simulink model "UPQC"  (R2021b)
settings: Solver=ode23tb  StartTime=0.0  StopTime=2.5  RelTol=1e-6  EnableMultiTasking=on
InitFcn:
  | Ts=20e-6;
undefined symbols (not defined in the file): DiscIntNeverNeededParam
libraries: spsIGBTDiodeLib x12, spsDiodeLib x6, spsSeriesRLCBranchLib x5, powerlib_extras x3, spsThreePhaseVIMeasurementLib x3, spsSaturableTransformerLib x3, spsThreePhaseSeriesRLCBranchLib x2, spsVoltageMeasurementLib x1, spsMultimeterLib x1, spsThreePhaseProgrammableVoltageSourceLib x1, spsGroundLib x1, spspowerguiLib x1
settings Model: Creator=srikanth  LastModifiedBy=B Sai Soumath
settings SolverCC: AlgebraicLoopSolver=LineSearch
settings DataIOCC: LimitDataPoints=on  SaveFormat=Array  SignalLoggingSaveFormat=ModelDataLogs  SaveOutput=off  SaveTime=off  ReturnWorkspaceOutputs=off
settings OptimizationCC: ExpressionDepthLimit=2147483647  LifeSpan=inf
settings DebuggingCC: AlgebraicLoopMsg=none  UnderspecifiedInitializationDetection=Classic  MergeDetectMultiDrivingBlocksExec=none  SolverPrmCheckMsg=warning  FcnCallInpInsideContextMsg=warning  StateNameClashWarn=warning  SFUnexpectedBacktrackingDiag=warning  SFNoUnconditionalDefaultTransitionDiag=warning  SFExecutionAtInitializationDiag=none  SFMachineParentedDataDiag=warning  ArithmeticOperatorsInVariantConditions=warning
settings HardwareCC: ProdBitPerPointer=32  ProdBitPerSizeT=32  ProdBitPerPtrDiffT=32  ProdLargestAtomicFloat=None  ProdIntDivRoundTo=Undefined  ProdEndianess=Unspecified  ProdWordSize=32  ProdHWDeviceType=32-bit Generic
settings ModelReferenceCC: PropagateSignalLabelsOutOfModel=off
settings SFSimCC: SimUseLocalCustomCode=off  CustomCodeUndefinedFunction=UseInterfaceOnly
settings RTWCC: RTWUseLocalCustomCode=off
settings CodeAppCC: StateflowObjectComments=on
settings GRTTargetCC: TargetLangStandard=C89/C90 (ANSI)  CombineOutputUpdateFcns=off  GRTInterface=on
settings ConfigComp: CovMetricSettings=dw  CovSaveCumulativeToWorkspaceVar=on  CovSaveSingleToWorkspaceVar=on  CovExternalEMLEnable=off

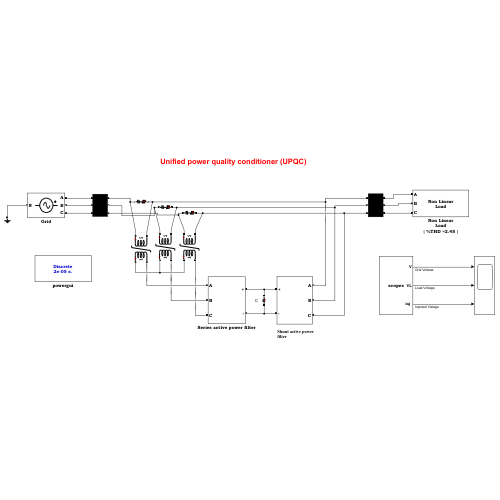
[thumbnail: Simulink's stored preview of the top-level diagram]
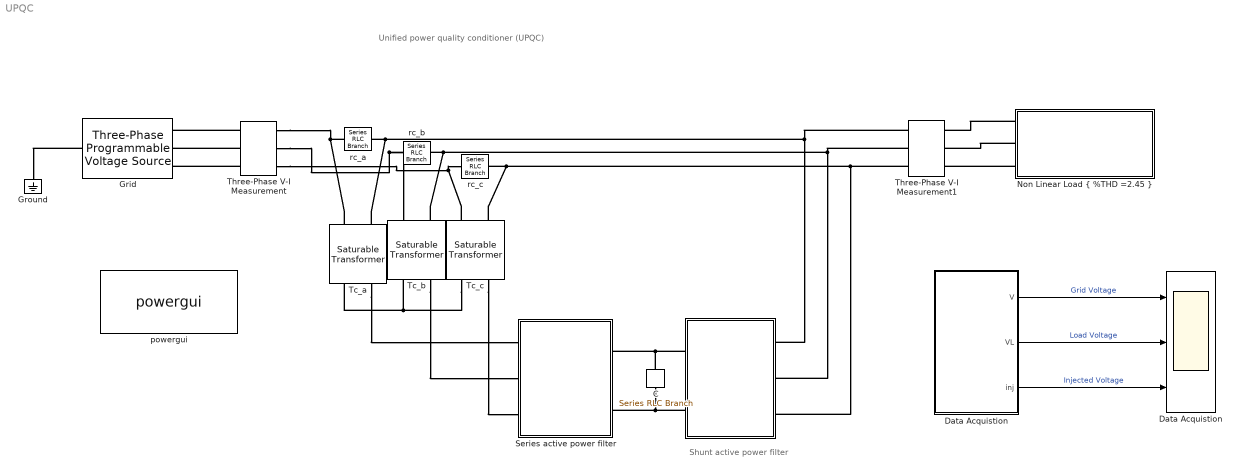
== system UPQC ==
  note: Shunt active power filter
  note: Unified power quality conditioner (UPQC)
  "                  " : Subsystem
  C : spsSeriesRLCBranchLib/Series RLC Branch  LConnTagsString=__new0  RConnTagsString=__new0  BranchType=C  Resistance=1  Inductance=1e-3  SetiL0=off  InitialCurrent=0  Capacitance=100e-6  Setx0=off  InitialVoltage=700  Measurements=None
  Data Acquistion : Scope  NumInputPorts=3
  Data Acquistion : Subsystem
      mask Display: fprintf('scopes')
  Grid : spsThreePhaseProgrammableVoltageSourceLib/Three-Phase Programmable Voltage Source  PositiveSequence="[400  0 50]"  VariationEntity=Amplitude  VariationType=Table of time-amplitude pairs  VariationTypeAlt=Step  VariationStep=0.5  VariationRate=10  VariationMagnitude=0.3  VariationFrequency=2  VariationTiming=[1 2]  VariationPhaseA=off  Amplitudes=[1 0.7 1 1.3 1]  TimeValues=[0 0.9 1 1.6 1.7]  HarmonicGeneration=on  HarmonicA=[5 0.2 0 2]  HarmonicB=[7 0.05 0 1]  Timing=[0.3 0.4]  BusType=swing  Pref=0  Qref=0  Qmin=-inf  Qmax=inf
  Ground : spsGroundLib/Ground  LConnTagsString=a
  "Non Linear Load { %THD =2.45 }" : Subsystem
      mask Display: fprintf('Non Linear\nLoad')
  Series active power filter : Subsystem
  Tc_a : spsSaturableTransformerLib/Saturable Transformer  ThreeWindings=off  Hysteresis=off  DataFile='hysteresis.mat'  Measurements=None  UNITS=pu  NominalPower=[4000 50]  Winding1="[380  0.02  0.02 ]"  Winding2="[380  0.02  0.02]"  Winding3="[ 315e3  0.002  0.08 ]"  Saturation=[ 0 0 ;1.016 9.043]*1e-3  CoreLoss=[117 0]  BreakLoop=off  DiscreteSolver=Trapezoidal iterative  DataType=off  InitialFlux=0  TransfoNumber=1
      settings: SourceProductBaseCode=PS
  Tc_b : spsSaturableTransformerLib/Saturable Transformer  ThreeWindings=off  Hysteresis=off  DataFile='hysteresis.mat'  Measurements=None  UNITS=pu  NominalPower=[4000 50]  Winding1="[380  0.02  0.02 ]"  Winding2="[380  0.02  0.02]"  Winding3="[ 315e3  0.002  0.08 ]"  Saturation=[ 0 0 ;1.016 9.043]*1e-3  CoreLoss=[117 0]  BreakLoop=off  DiscreteSolver=Trapezoidal iterative  DataType=off  InitialFlux=0  TransfoNumber=1
      settings: SourceProductBaseCode=PS
  Tc_c : spsSaturableTransformerLib/Saturable Transformer  ThreeWindings=off  Hysteresis=off  DataFile='hysteresis.mat'  Measurements=None  UNITS=pu  NominalPower=[4000 50]  Winding1="[380  0.02  0.02 ]"  Winding2="[380  0.02  0.02]"  Winding3="[ 315e3  0.002  0.08 ]"  Saturation=[ 0 0 ;1.016 9.043]*1e-3  CoreLoss=[117 0]  BreakLoop=off  DiscreteSolver=Trapezoidal iterative  DataType=off  InitialFlux=0  TransfoNumber=1
      settings: SourceProductBaseCode=PS
  Three-Phase V-I Measurement : spsThreePhaseVIMeasurementLib/Three-Phase V-I Measurement  VoltageMeasurement=phase-to-ground  SetLabelV=on  LabelV=Vabc  Vpu=off  VpuLL=off  CurrentMeasurement=yes  SetLabelI=on  LabelI=Iabc  Ipu=off  Pbase=100e6  Vbase=500e3  OutputType=Complex  PhasorSimulation=off  PSBequivalent=0
  Three-Phase V-I Measurement1 : spsThreePhaseVIMeasurementLib/Three-Phase V-I Measurement  VoltageMeasurement=phase-to-ground  SetLabelV=on  LabelV=V_L  Vpu=off  VpuLL=off  CurrentMeasurement=yes  SetLabelI=on  LabelI=I_L  Ipu=off  Pbase=100e6  Vbase=500e3  OutputType=Complex  PhasorSimulation=off  PSBequivalent=0
  powergui : spspowerguiLib/powergui  Priority=1  SimulationMode=Discrete  SampleTime=Ts  frequency=60  Iterations=50  frequencyindice=50  Pbase=100e6  ErrMax=1e-4  UnitsV=kV  UnitsW=MW  buscounter=0  FunctionMessages=off  echomessages=off  EnableUseOfTLC=off  CurrentSourceSwitches=off  DisableSnubberDevices=off  DisableRonSwitches=off  DisableVfSwitches=off  DisplayEquations=off  AutomaticDiscreteSolvers=off  SolverType=Tustin/Backward Euler (TBE)  Interpol=off  ExternalGateDelay=off  methode=off  Ts=0  x0status=blocks  SPID=off  SwTol=0  HookPort=off  NonlinearTolerance=1e-4  nMaxIteration=100  ContinueOnMaxIteration=off  RestoreLinks=warning  ResistiveCurrentMeasurement=off  Frange=[0:2:500]  Ylog=off  Xlog=on  ShowGrid=off  save=off  variable=ZData  structure=Grid_pi  ZoomFFT=on  StartTime=0.9  cycles=1  DisplayStyle=3  fundamental=50  FreqAxis=on  MaxFrequency=2500  frequencyindicesteady=1  RmsSteady=1  display=off
  rc_a : spsSeriesRLCBranchLib/Series RLC Branch  LConnTagsString=__new0  RConnTagsString=__new0  BranchType=RC  Resistance=1  Inductance=1e-3  SetiL0=off  InitialCurrent=0  Capacitance=100e-6  Setx0=off  InitialVoltage=0  Measurements=Branch voltage
  rc_b : spsSeriesRLCBranchLib/Series RLC Branch  LConnTagsString=__new0  RConnTagsString=__new0  BranchType=RC  Resistance=1  Inductance=1e-3  SetiL0=off  InitialCurrent=0  Capacitance=100e-6  Setx0=off  InitialVoltage=0  Measurements=Branch voltage
  rc_c : spsSeriesRLCBranchLib/Series RLC Branch  LConnTagsString=__new0  RConnTagsString=__new0  BranchType=RC  Resistance=1  Inductance=1e-3  SetiL0=off  InitialCurrent=0  Capacitance=100e-6  Setx0=off  InitialVoltage=0  Measurements=Branch voltage
  wires:
  Data Acquistion/1(V) -> Data Acquistion/1  "Grid Voltage"
  Data Acquistion/2(VL) -> Data Acquistion/2  "Load Voltage"
  Data Acquistion/3("inj ") -> Data Acquistion/3  "Injected Voltage"
  connections:
  Grid/LConn1 -- Ground/LConn1
  Three-Phase V-I Measurement/LConn1 -- Grid/RConn1
  Three-Phase V-I Measurement/LConn2 -- Grid/RConn2
  Three-Phase V-I Measurement/LConn3 -- Grid/RConn3
  rc_a/RConn1 -- Three-Phase V-I Measurement/RConn1 -- Tc_a/RConn1
  rc_b/RConn1 -- Three-Phase V-I Measurement/RConn2 -- Tc_b/RConn1
  Three-Phase V-I Measurement/RConn3 -- rc_c/RConn1 -- Tc_c/RConn1
  Tc_a/LConn2 -- Series active power filter/LConn1
  Tc_b/LConn2 -- Series active power filter/LConn2
  Tc_c/LConn2 -- Series active power filter/LConn3
  Tc_c/LConn1 -- Tc_a/LConn1 -- Tc_b/LConn1
  "                  "/RConn2 -- C/RConn1 -- Series active power filter/RConn2
  Three-Phase V-I Measurement1/LConn3 -- "                  "/LConn3 -- Tc_c/RConn2 -- rc_c/LConn1
  Three-Phase V-I Measurement1/LConn2 -- "                  "/LConn2 -- Tc_b/RConn2 -- rc_b/LConn1
  Three-Phase V-I Measurement1/LConn1 -- "                  "/LConn1 -- Tc_a/RConn2 -- rc_a/LConn1
  "                  "/RConn1 -- C/LConn1 -- Series active power filter/RConn1
  "Non Linear Load { %THD =2.45 }"/LConn1 -- Three-Phase V-I Measurement1/RConn1
  "Non Linear Load { %THD =2.45 }"/LConn2 -- Three-Phase V-I Measurement1/RConn2
  "Non Linear Load { %THD =2.45 }"/LConn3 -- Three-Phase V-I Measurement1/RConn3

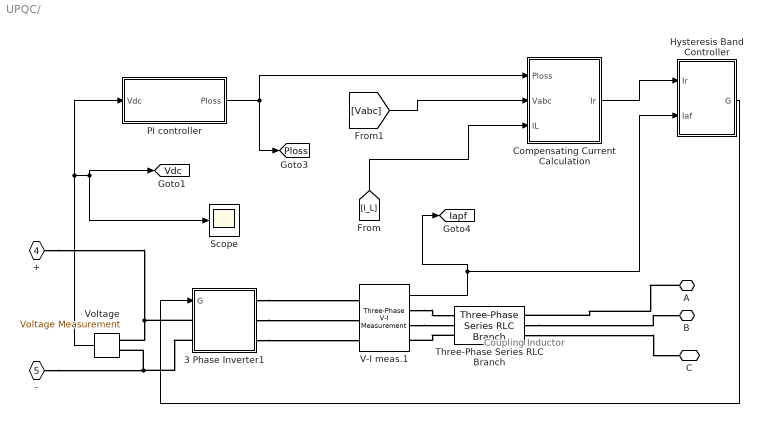
== system UPQC/                   ==
  note: Coupling Inductor
  3 Phase Inverter1 : Subsystem
  Compensating Current Calculation : Subsystem
  Hysteresis Band Controller : Subsystem
  PI controller : Subsystem
  Scope : Scope
  Three-Phase Series RLC Branch : spsThreePhaseSeriesRLCBranchLib/Three-Phase Series RLC Branch  LConnTagsString=A|B|C  RConnTagsString=A|B|C  BranchType=L  Resistance=0.0001  Inductance=10e-3  Capacitance=.2e-3  Measurements=None
  V-I meas.1 : spsThreePhaseVIMeasurementLib/Three-Phase V-I Measurement  VoltageMeasurement=phase-to-ground  SetLabelV=on  LabelV=Vnm  Vpu=off  VpuLL=off  CurrentMeasurement=yes  SetLabelI=off  LabelI=Iabc  Ipu=off  Pbase=100e6  Vbase=500e3  OutputType=Complex  PhasorSimulation=off  PSBequivalent=0
  Voltage : spsVoltageMeasurementLib/Voltage Measurement  PhasorSimulation=off  OutputType=Complex  PSBequivalent=0
  A : PMIOPort  Side=Left
  B : PMIOPort  Port=2  Side=Left
  C : PMIOPort  Port=3  Side=Left
  + : PMIOPort  Tag=PMCPort  Port=4  Side=Right
  - : PMIOPort  Tag=PMCPort  Port=5  Side=Right
  tag scope: Iapf=global, Ploss=global, Vdc=global
  wires:
  V-I meas.1/1 -> Hysteresis Band Controller/2(Iaf), [Iapf]
  Voltage/1 -> PI controller/1(Vdc), Scope/1, [Vdc]
  [I_L] -> Compensating Current Calculation/3(IL)
  [Vabc] -> Compensating Current Calculation/2(Vabc)
  Compensating Current Calculation/1(Ir) -> Hysteresis Band Controller/1(Ir)
  PI controller/1(Ploss) -> [Ploss], Compensating Current Calculation/1(Ploss)
  Hysteresis Band Controller/1(G) -> 3 Phase Inverter1/1(G)
  connections:
  +/RConn1 -- 3 Phase Inverter1/LConn1 -- Voltage/LConn1
  3 Phase Inverter1/RConn1 -- V-I meas.1/LConn1
  3 Phase Inverter1/RConn2 -- V-I meas.1/LConn2
  Three-Phase Series RLC Branch/LConn3 -- V-I meas.1/RConn3
  V-I meas.1/RConn2 -- Three-Phase Series RLC Branch/LConn2
  3 Phase Inverter1/RConn3 -- V-I meas.1/LConn3
  V-I meas.1/RConn1 -- Three-Phase Series RLC Branch/LConn1
  A/RConn1 -- Three-Phase Series RLC Branch/RConn1
  Three-Phase Series RLC Branch/RConn2 -- B/RConn1
  Three-Phase Series RLC Branch/RConn3 -- C/RConn1
  -/RConn1 -- 3 Phase Inverter1/LConn2 -- Voltage/LConn2

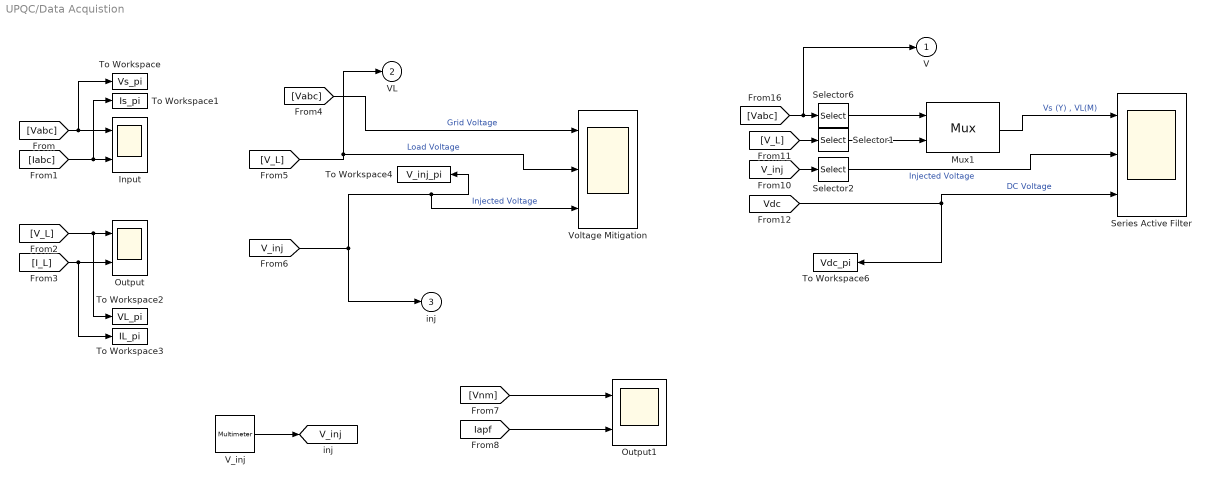
== system UPQC/Data Acquistion ==
  Input : Scope  NumInputPorts=2
  Mux1 : Mux  Inputs=2
      settings: DisplayOption=signals
  Output : Scope  NumInputPorts=2
  Output1 : Scope  NumInputPorts=2
  Selector1 : Selector  InputPortWidth=3  IndexOptions=Index vector (dialog)  Indices=1  OutputSizes=1
  Selector2 : Selector  InputPortWidth=3  IndexOptions=Index vector (dialog)  Indices=1  OutputSizes=1
  Selector6 : Selector  InputPortWidth=3  IndexOptions=Index vector (dialog)  Indices=1  OutputSizes=1
  Series Active Filter : Scope  NumInputPorts=3
  To Workspace : ToWorkspace  VariableName=Vs_pi  SampleTime=Ts
  To Workspace1 : ToWorkspace  VariableName=Is_pi  SampleTime=Ts
  To Workspace2 : ToWorkspace  VariableName=VL_pi  SampleTime=Ts
  To Workspace3 : ToWorkspace  VariableName=IL_pi  SampleTime=Ts
  To Workspace4 : ToWorkspace  VariableName=V_inj_pi  SampleTime=Ts
  To Workspace6 : ToWorkspace  VariableName=Vdc_pi  SampleTime=Ts
  V_inj : spsMultimeterLib/Multimeter  PhasorSimulation=off  OutputType=Complex  sel=[1 2 3]  L=3  Gain=[1 1 1]  yselected={'Ub: rc_a','Ub: rc_b','Ub: rc_c'};  PSBOutputType=1  PSBequivalent=0  AxesSetting=[0,0.1,-100,100]  Display=0  SavedBlockNames=-11
  Voltage Mitigation : Scope  NumInputPorts=3
  V : Outport  VectorParamsAs1DForOutWhenUnconnected=off
  VL : Outport  Port=2  VectorParamsAs1DForOutWhenUnconnected=off
  "inj " : Outport  Port=3  VectorParamsAs1DForOutWhenUnconnected=off
  tag scope: V_inj=global
  wires:
  [Vabc] -> Input/1, To Workspace/1
  [Iabc] -> Input/2, To Workspace1/1
  [V_L] -> Output/1, To Workspace2/1
  [I_L] -> Output/2, To Workspace3/1
  [Vabc] -> Voltage Mitigation/1  "Grid Voltage"
  [V_L] -> Voltage Mitigation/2, VL/1  "Load Voltage"
  [V_inj] -> Voltage Mitigation/3, To Workspace4/1, "inj "/1  "Injected Voltage"
  [V_L] -> Selector1/1
  [V_inj] -> Selector2/1
  [Vdc] -> Series Active Filter/3, To Workspace6/1  "DC Voltage"
  Selector2/1 -> Series Active Filter/2  "Injected Voltage"
  [Vabc] -> Selector6/1, V/1
  Selector1/1 -> Mux1/2
  Mux1/1 -> Series Active Filter/1  "Vs (Y) , VL(M)"
  Selector6/1 -> Mux1/1
  V_inj/1 -> [V_inj]
  [Iapf] -> Output1/2
  [Vnm] -> Output1/1

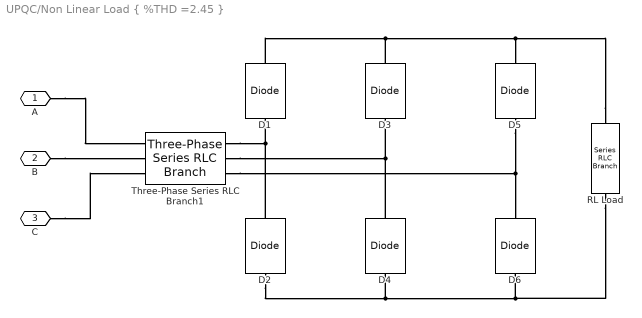
== system UPQC/Non Linear Load { %THD =2.45 } ==
  D{1..6} (6 alike) : spsDiodeLib/Diode  Ron=0.001  Lon=0  Vf=0.8  IC=0  UseSnubber=off  Rs=500  Cs=250e-9  Measurements=off
  RL Load : spsSeriesRLCBranchLib/Series RLC Branch  LConnTagsString=__new0  RConnTagsString=__new0  BranchType=RL  Resistance=60  Inductance=0.15e-3  SetiL0=off  InitialCurrent=0  Capacitance=1e-6  Setx0=off  InitialVoltage=0  Measurements=None
  Three-Phase Series RLC Branch1 : spsThreePhaseSeriesRLCBranchLib/Three-Phase Series RLC Branch  LConnTagsString=A|B|C  RConnTagsString=A|B|C  BranchType=RL  Resistance=0.4  Inductance=15e-3  Capacitance=1e-6  Measurements=None
  A : PMIOPort  Side=Left
  B : PMIOPort  Port=2  Side=Left
  C : PMIOPort  Port=3  Side=Left
  connections:
  C/RConn1 -- Three-Phase Series RLC Branch1/LConn3
  B/RConn1 -- Three-Phase Series RLC Branch1/LConn2
  A/RConn1 -- Three-Phase Series RLC Branch1/LConn1
  Three-Phase Series RLC Branch1/RConn3 -- D6/RConn1 -- D5/LConn1
  Three-Phase Series RLC Branch1/RConn2 -- D4/RConn1 -- D3/LConn1
  RL Load/RConn1 -- D6/LConn1 -- D4/LConn1 -- D2/LConn1
  RL Load/LConn1 -- D5/RConn1 -- D3/RConn1 -- D1/RConn1
  Three-Phase Series RLC Branch1/RConn1 -- D2/RConn1 -- D1/LConn1

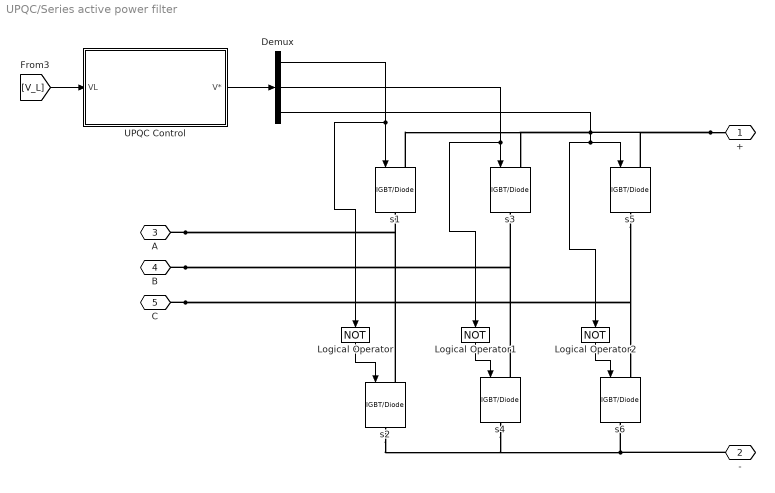
== system UPQC/Series active power filter ==
  Demux : Demux  Outputs=3
      settings: DisplayOption=none
  Logical Operator : Logic  Operator=NOT  AllPortsSameDT=off  OutDataTypeStr=boolean
  Logical Operator1 : Logic  Operator=NOT  AllPortsSameDT=off  OutDataTypeStr=boolean
  Logical Operator2 : Logic  Operator=NOT  AllPortsSameDT=off  OutDataTypeStr=boolean
  UPQC Control : Subsystem
      mask Display: fprintf('Series\nFilter')
  s{1..6} (6 alike) : spsIGBTDiodeLib/IGBT//Diode  Ron=1e-3  Rs=1e5  Cs=inf  Measurements=off
  + : PMIOPort  Side=Right
  - : PMIOPort  Port=2  Side=Right
  A : PMIOPort  Port=3  Side=Left
  B : PMIOPort  Port=4  Side=Left
  C : PMIOPort  Port=5  Side=Left
  wires:
  Demux/2 -> s3/1, Logical Operator1/1
  Demux/1 -> s1/1, Logical Operator/1
  Logical Operator/1 -> s2/1
  Logical Operator1/1 -> s4/1
  Logical Operator2/1 -> s6/1
  Demux/3 -> Logical Operator2/1, s5/1
  UPQC Control/1(V*) -> Demux/1
  [V_L] -> UPQC Control/1(VL)
  connections:
  +/RConn1 -- s5/LConn1 -- s1/LConn1 -- s3/LConn1
  A/RConn1 -- s1/RConn1 -- s2/LConn1
  -/RConn1 -- s6/RConn1 -- s4/RConn1 -- s2/RConn1
  B/RConn1 -- s3/RConn1 -- s4/LConn1
  C/RConn1 -- s5/RConn1 -- s6/LConn1

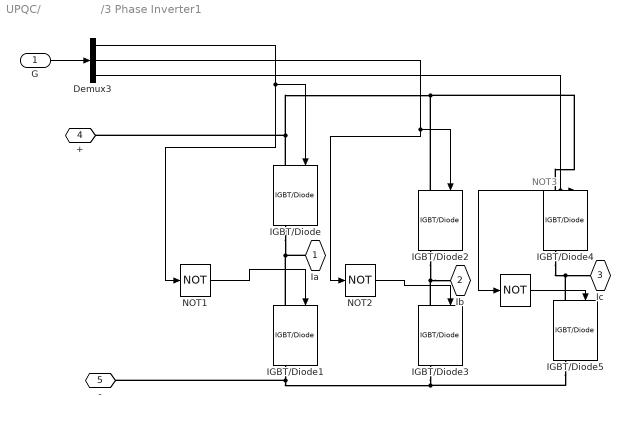
== system UPQC/                  /3 Phase Inverter1 ==
  note: NOT3
  G : Inport
  " " : Logic  Operator=NOT  AllPortsSameDT=off  OutDataTypeStr=boolean
  Demux3 : Demux  Outputs=3
  IGBT/Diode{,1..5} (6 alike) : spsIGBTDiodeLib/IGBT//Diode  Ron=1e-3  Rs=1e5  Cs=inf  Measurements=on
  NOT1 : Logic  Operator=NOT  AllPortsSameDT=off  OutDataTypeStr=boolean
  NOT2 : Logic  Operator=NOT  AllPortsSameDT=off  OutDataTypeStr=boolean
  Ia : PMIOPort  Side=Right
  Ib : PMIOPort  Port=2  Side=Right
  Ic : PMIOPort  Port=3  Side=Right
  + : PMIOPort  Port=4  Side=Left
  - : PMIOPort  Port=5  Side=Left
  wires:
  G/1 -> Demux3/1
  Demux3/3 -> IGBT/Diode4/1, " "/1
  Demux3/2 -> NOT2/1, IGBT/Diode2/1
  Demux3/1 -> NOT1/1, IGBT/Diode/1
  " "/1 -> IGBT/Diode5/1
  NOT2/1 -> IGBT/Diode3/1
  NOT1/1 -> IGBT/Diode1/1
  connections:
  IGBT/Diode4/RConn1 -- Ic/RConn1 -- IGBT/Diode5/LConn1
  -/RConn1 -- IGBT/Diode5/RConn1 -- IGBT/Diode3/RConn1 -- IGBT/Diode1/RConn1
  Ib/RConn1 -- IGBT/Diode3/LConn1 -- IGBT/Diode2/RConn1
  +/RConn1 -- IGBT/Diode4/LConn1 -- IGBT/Diode2/LConn1 -- IGBT/Diode/LConn1
  Ia/RConn1 -- IGBT/Diode1/LConn1 -- IGBT/Diode/RConn1

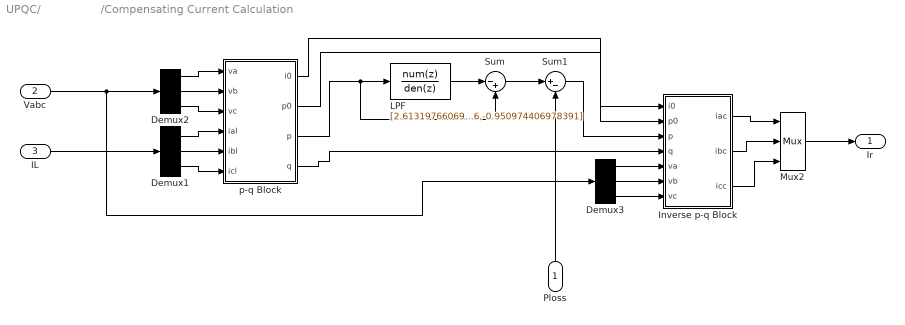
== system UPQC/                  /Compensating Current Calculation ==
  Ploss : Inport
  Vabc : Inport  Port=2
  IL : Inport  Port=3
  Demux1 : Demux  Outputs=3
  Demux2 : Demux  Outputs=3
  Demux3 : Demux  Outputs=3
  Inverse p-q Block : MATLAB Function  TreatAsAtomicUnit=on
  LPF : DiscreteFilter  Numerator=[2.61319766069688e-06,1.03220890220108e-05,2.54833591692978e-06]  Denominator=[1,-2.94973451762717,2.90072440822816,-0.950974406978391]  InitialDenominatorStates=1  SampleTime=1/(5e3)
  Mux2 : Mux  Inputs=3
  Sum : Sum  Inputs=|-+
  Sum1 : Sum  Inputs=|+-
  p-q Block : MATLAB Function  TreatAsAtomicUnit=on
  Ir : Outport  VectorParamsAs1DForOutWhenUnconnected=off
  wires:
  Inverse p-q Block/3(icc) -> Mux2/3
  IL/1 -> Demux1/1
  Demux1/2 -> p-q Block/5(ibl)
  Mux2/1 -> Ir/1
  Inverse p-q Block/1(iac) -> Mux2/1
  Demux1/1 -> p-q Block/4(ial)
  Inverse p-q Block/2(ibc) -> Mux2/2
  p-q Block/1(i0) -> Inverse p-q Block/1(i0)
  p-q Block/3(p) -> LPF/1, Sum/2
  Ploss/1 -> Sum1/2
  LPF/1 -> Sum/1
  Sum/1 -> Sum1/1
  Sum1/1 -> Inverse p-q Block/3(p)
  p-q Block/4(q) -> Inverse p-q Block/4(q)
  Demux1/3 -> p-q Block/6(icl)
  p-q Block/2(p0) -> Inverse p-q Block/2(p0)
  Demux2/3 -> p-q Block/3(vc)
  Demux2/2 -> p-q Block/2(vb)
  Demux2/1 -> p-q Block/1(va)
  Vabc/1 -> Demux2/1, Demux3/1
  Demux3/1 -> Inverse p-q Block/5(va)
  Demux3/2 -> Inverse p-q Block/6(vb)
  Demux3/3 -> Inverse p-q Block/7(vc)

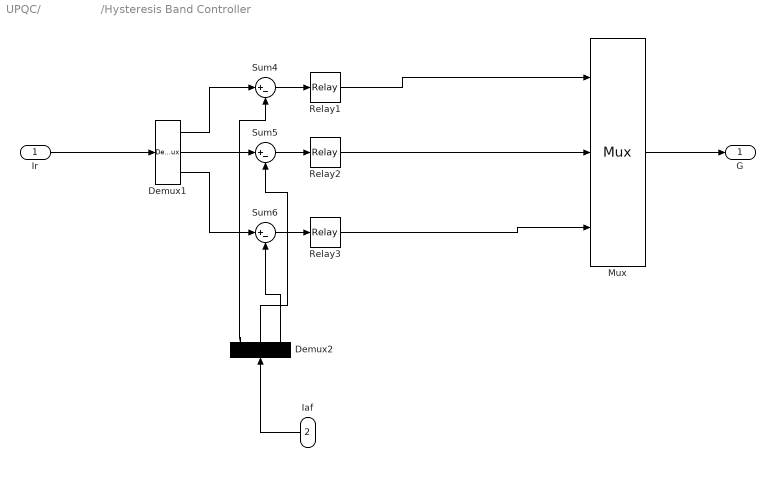
== system UPQC/                  /Hysteresis Band Controller ==
  Ir : Inport
  Iaf : Inport  Port=2
  Demux1 : Demux  Outputs=3
  Demux2 : Demux  Outputs=3
  Mux : Mux  Inputs=3
  Relay1 : Relay  OnSwitchValue=0.01  OffSwitchValue=-0.01  OutDataTypeStr=boolean  ZeroCross=off
  Relay2 : Relay  OnSwitchValue=0.01  OffSwitchValue=-0.01  OutDataTypeStr=boolean  ZeroCross=off
  Relay3 : Relay  OnSwitchValue=0.01  OffSwitchValue=-0.01  OutDataTypeStr=boolean  ZeroCross=off
  Sum4 : Sum  Inputs=|+-
  Sum5 : Sum  Inputs=|+-
  Sum6 : Sum  Inputs=|+-
  G : Outport  VectorParamsAs1DForOutWhenUnconnected=off
  wires:
  Demux2/2 -> Sum5/2
  Demux1/2 -> Sum5/1
  Sum6/1 -> Relay3/1
  Demux1/1 -> Sum4/1
  Demux1/3 -> Sum6/1
  Demux2/3 -> Sum6/2
  Sum5/1 -> Relay2/1
  Demux2/1 -> Sum4/2
  Sum4/1 -> Relay1/1
  Ir/1 -> Demux1/1
  Iaf/1 -> Demux2/1
  Mux/1 -> G/1
  Relay1/1 -> Mux/1
  Relay3/1 -> Mux/3
  Relay2/1 -> Mux/2

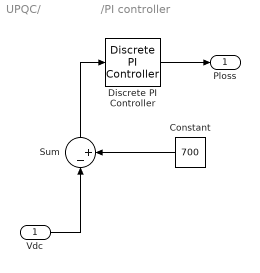
== system UPQC/                  /PI controller ==
  Vdc : Inport
  Constant : Constant  Value=700
  Discrete PI Controller : powerlib_extras/Discrete  Control Blocks/Discrete PI Controller  Kp=10  Ki=0.1  Par_Limits=[1e6 -1e6]  Init=0  Ts=5e-6
  Sum : Sum  Inputs=|-+
  Ploss : Outport  VectorParamsAs1DForOutWhenUnconnected=off
  wires:
  Constant/1 -> Sum/2
  Sum/1 -> Discrete PI Controller/1
  Discrete PI Controller/1 -> Ploss/1
  Vdc/1 -> Sum/1

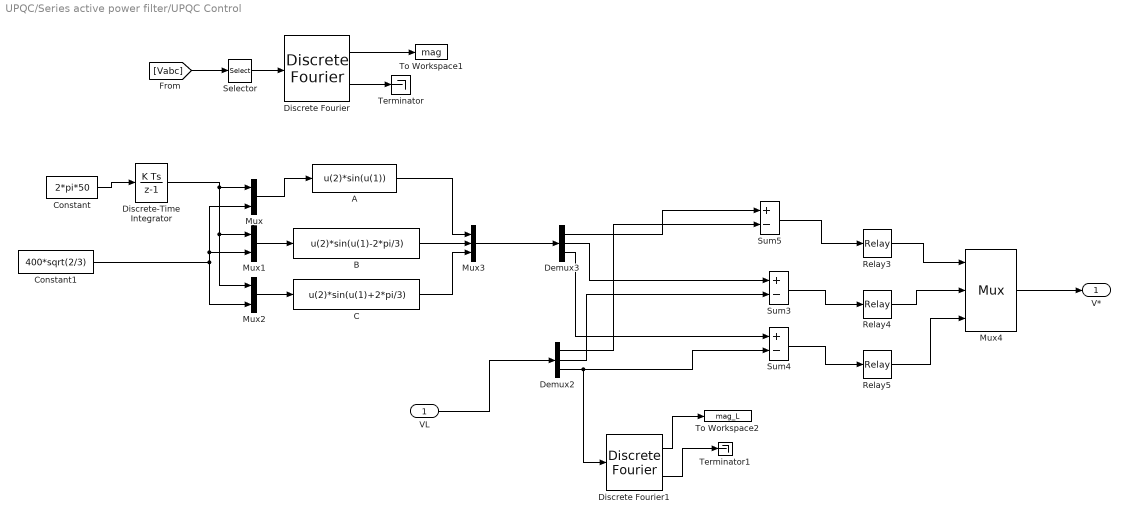
== system UPQC/Series active power filter/UPQC Control ==
  VL : Inport
  A : Fcn  Expr=u(2)*sin(u(1))
  B : Fcn  Expr=u(2)*sin(u(1)-2*pi/3)
  C : Fcn  Expr=u(2)*sin(u(1)+2*pi/3)
  Constant : Constant  Value=2*pi*50
  Constant1 : Constant  Value=400*sqrt(2/3)
  Demux2 : Demux  Outputs=3
  Demux3 : Demux  Outputs=3
  Discrete Fourier : powerlib_extras/Discrete Measurements/Discrete  Fourier  Freq=50  n=1  Par_Init=[0 0]  Ts=Ts
      settings: SourceProductBaseCode=PS
  Discrete Fourier1 : powerlib_extras/Discrete Measurements/Discrete  Fourier  Freq=50  n=1  Par_Init=[0 0]  Ts=Ts
      settings: SourceProductBaseCode=PS
  Discrete-Time Integrator : DiscreteIntegrator  SampleTime=Ts  ICPrevOutput=DiscIntNeverNeededParam  ICPrevScaledInput=DiscIntNeverNeededParam
  Mux : Mux  Inputs=2
  Mux1 : Mux  Inputs=2
  Mux2 : Mux  Inputs=2
  Mux3 : Mux  Inputs=3
  Mux4 : Mux  Inputs=3
  Relay3 : Relay  OnSwitchValue=1  OffSwitchValue=-1
  Relay4 : Relay  OnSwitchValue=1  OffSwitchValue=-1
  Relay5 : Relay  OnSwitchValue=1  OffSwitchValue=-1
  Selector : Selector  InputPortWidth=3  IndexOptions=Index vector (dialog)  Indices=1  OutputSizes=1
  Sum3 : Sum  Inputs=+-
  Sum4 : Sum  Inputs=+-
  Sum5 : Sum  Inputs=+-
  Terminator : Terminator
  Terminator1 : Terminator
  To Workspace1 : ToWorkspace  VariableName=mag  SampleTime=Ts
  To Workspace2 : ToWorkspace  VariableName=mag_L  SampleTime=Ts
  V* : Outport  VectorParamsAs1DForOutWhenUnconnected=off
  wires:
  Constant/1 -> Discrete-Time Integrator/1
  Discrete-Time Integrator/1 -> Mux/1, Mux2/1, Mux1/1
  Constant1/1 -> Mux1/2, Mux/2, Mux2/2
  Mux/1 -> A/1
  Mux1/1 -> B/1
  Mux2/1 -> C/1
  Discrete Fourier/2 -> Terminator/1
  Selector/1 -> Discrete Fourier/1
  [Vabc] -> Selector/1
  Discrete Fourier/1 -> To Workspace1/1
  A/1 -> Mux3/1
  B/1 -> Mux3/2
  C/1 -> Mux3/3
  Discrete Fourier1/2 -> Terminator1/1
  Sum5/1 -> Relay3/1
  Sum3/1 -> Relay4/1
  Sum4/1 -> Relay5/1
  Relay3/1 -> Mux4/1
  Relay4/1 -> Mux4/2
  Relay5/1 -> Mux4/3
  Mux4/1 -> V*/1
  Discrete Fourier1/1 -> To Workspace2/1
  VL/1 -> Demux2/1
  Demux3/1 -> Sum5/1
  Demux2/3 -> Sum4/2, Discrete Fourier1/1
  Demux2/1 -> Sum5/2
  Demux3/3 -> Sum4/1
  Demux2/2 -> Sum3/2
  Demux3/2 -> Sum3/1
  Mux3/1 -> Demux3/1

== matlab function UPQC/                  /Compensating Current Calculation/Inverse p-q Block ==
  data: i0 input; p0 input; p input; iac output; q input; va input; vb input; vc input; ibc output; icc output
function [iac,ibc,icc]= fcn(i0,p0,p,q,va,vb,vc)
%#codegen
v_zero=(va+vb+vc)/sqrt(3);
v_alpha=(va-vb/2-vc/2)*sqrt(2/3);
v_beta=(vb-vc)/sqrt(2);
i_zero=i0;
i_alpha=(v_alpha.*p+v_beta.*q)/(v_alpha.^2+v_beta.^2);
i_beta=(v_beta.*p-v_alpha.*q)/(v_alpha.^2+v_beta.^2);
iac=sqrt(2/3)*(i_zero/sqrt(2)+i_alpha);
ibc=sqrt(2/3)*(i_zero./sqrt(2)-i_alpha/2+sqrt(3)*i_beta/2);
icc=sqrt(2/3)*(i_zero./sqrt(2)-i_alpha/2-i_beta*sqrt(3)/2);

== matlab function UPQC/                  /Compensating Current Calculation/p-q Block ==
  data: i0 output; p0 output; va input; p output; vb input; vc input; ial input; ibl input; icl input; q output
function [i0,p0,p,q]= fcn(va,vb,vc,ial,ibl,icl)
%#codegen
v_zero=(va+vb+vc)/sqrt(3);
v_alpha=(va-vb/2-vc/2)*sqrt(2/3);
v_beta=(vb-vc)/sqrt(2);
il_zero=(ial+ibl+icl)/sqrt(3);
il_alpha=(ial-ibl/2-icl/2)*sqrt(2/3);
il_beta=(ibl-icl)/sqrt(2);
i0=il_zero;
p0=v_zero.*il_zero;
p=v_alpha.*il_alpha+v_beta.*il_beta;
q=v_beta.*il_alpha-v_alpha.*il_beta;
